simulink model "simula"  (R2021a)
settings: Solver=VariableStepAuto  StartTime=0.0  StopTime=5  RelTol=1e-3
values from neighbouring files (symbols this model uses):
  B = 1145    [simu.m]
  Kr = 102000    [simu.m]
  Ks = 8090    [simu.m]
  Mc = 253    [simu.m]
  Mr = 26    [simu.m]
settings Model: Creator=HIGOR  LastModifiedBy=HIGOR

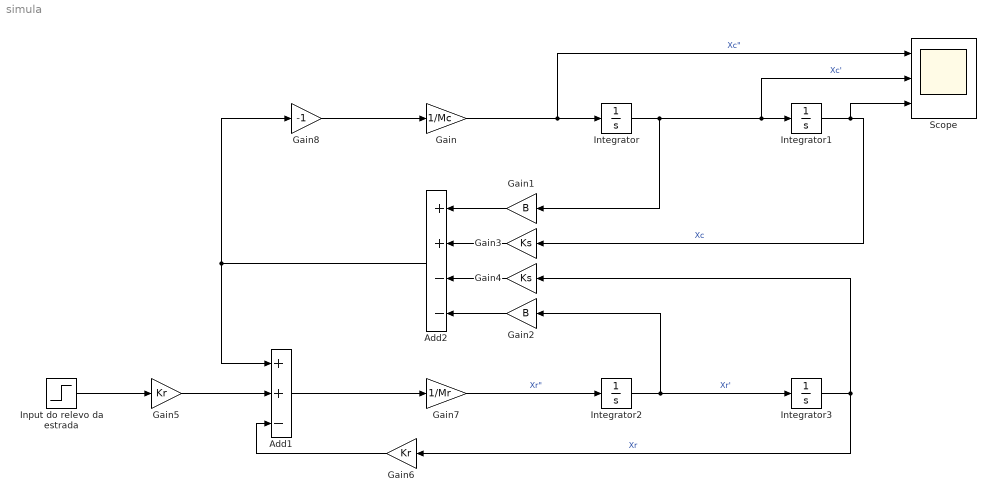
== system simula ==
  Add1 : Sum  Inputs=++-
  Add2 : Sum  Inputs=++--
  Gain : Gain  Gain=1/Mc
  Gain1 : Gain  Gain=B
  Gain2 : Gain  Gain=B
  Gain3 : Gain  Gain=Ks
  Gain4 : Gain  Gain=Ks
  Gain5 : Gain  Gain=Kr
  Gain6 : Gain  Gain=Kr
  Gain7 : Gain  Gain=1/Mr
  Gain8 : Gain  Gain=-1
  Input do relevo da estrada : Step  SampleTime=0
  Integrator{,1..3} (4 alike) : Integrator
  Scope : Scope  NumInputPorts=3
  wires:
  Integrator/1 -> Gain1/1, Scope/2, Integrator1/1  "Xc'"
  Gain/1 -> Scope/1, Integrator/1  "Xc\""
  Gain7/1 -> Integrator2/1  "Xr\""
  Integrator2/1 -> Gain2/1, Integrator3/1  "Xr'"
  Gain1/1 -> Add2/1
  Gain2/1 -> Add2/4
  Gain3/1 -> Add2/2
  Gain4/1 -> Add2/3
  Gain8/1 -> Gain/1
  Add1/1 -> Gain7/1
  Integrator1/1 -> Scope/3, Gain3/1  "Xc"
  Integrator3/1 -> Gain6/1, Gain4/1  "Xr"
  Add2/1 -> Gain8/1, Add1/1
  Gain5/1 -> Add1/2
  Gain6/1 -> Add1/3
  Input do relevo da estrada/1 -> Gain5/1
